simulink model "zadacha_03_model"  (Simulink 7.1)
settings: Solver=ode45  StartTime=0.0  StopTime=100  RelTol=1e-3
values from neighbouring files (symbols this model uses):
  D = fp(3)    [pidfunc.m]
  I = fp(2)    [pidfunc.m]
  P = fp(1)    [pidfunc.m]
libraries: simulink_extras x1
settings Model: Creator=Slavi  LastModifiedBy=Slavi

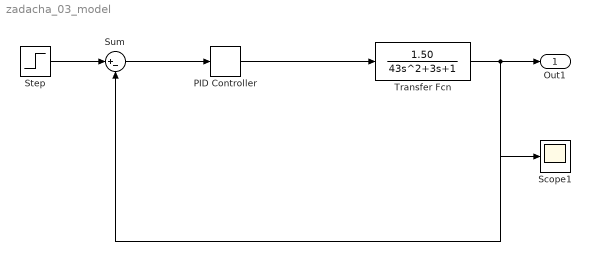
== system zadacha_03_model ==
  PID Controller : simulink_extras/Additional Linear/PID Controller  SystemSampleTime=-1  P=P  I=I  D=D
  Scope1 : Scope
  Step : Step  Time=0
  Sum : Sum  Inputs=|+-  OutDataType=sfix(16)  OutScaling=2^0
  Transfer Fcn : TransferFcn  Numerator=[1.50]  Denominator=[43 3 1]
  Out1 : Outport  OutDataType=sfix(16)  OutScaling=2^0
  wires:
  Transfer Fcn/1 -> Out1/1, Scope1/1, Sum/2
  Step/1 -> Sum/1
  Sum/1 -> PID Controller/1
  PID Controller/1 -> Transfer Fcn/1
